simulink model "amplifierboard"  (R2020b)
settings: Solver=FixedStepDiscrete  StartTime=0.0  StopTime=2  FixedStep=0.01  RelTol=1e-3
InitFcn:
  | mbd_s32k_consistency_checks(bdroot(gcs));
undefined symbols (not defined in the file): AutoLowerVal, AutoRaiseVal, HoldVal, LED_En, LED_Off, LED_On, Logic_High, Logic_Low, LQFP, ManualLowerVal, ManualRaiseVal, PWRWNDW_CHDLCK, sC_bool_PWMEN, sC_cnt_FWSetting, sC_cnt_Mtr_DrvNo_HB, sC_cnt_PWMHB1to4, sC_cnt_PWMHB5to8, sC_cnt_TargetSlowRange, sC_pct_ManualMax, sC_pct_RampDwn, sC_pct_RampUp, sC_pct_StartPWM, sC_pct_Targetmax, SwitchPackRangeOffset, Threshold_Value, Tolerant_Time
libraries: mbd_s32k1xx_ec_toolbox x205, simulink x59, canmsglib x19, Filter x15, wndwcmd x3
(part 2 of 6)

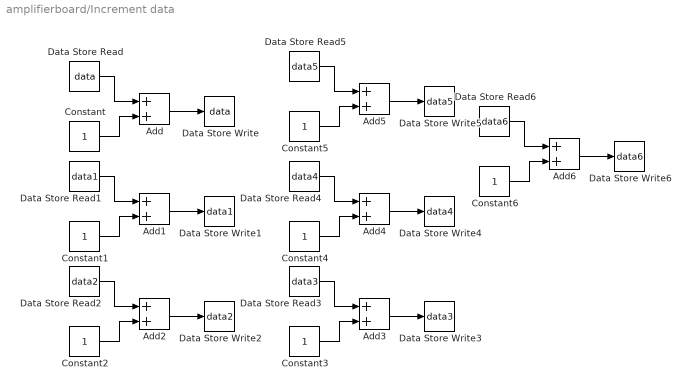
== system amplifierboard/Increment data ==
  Add{,1..6} (7 alike) : Sum
  Constant{,1..6} (7 alike) : Constant  OutDataTypeStr=uint8
  Data Store Read : DataStoreRead  DataStoreName=data
  Data Store Read1 : DataStoreRead  DataStoreName=data1
  Data Store Read2 : DataStoreRead  DataStoreName=data2
  Data Store Read3 : DataStoreRead  DataStoreName=data3
  Data Store Read4 : DataStoreRead  DataStoreName=data4
  Data Store Read5 : DataStoreRead  DataStoreName=data5
  Data Store Read6 : DataStoreRead  DataStoreName=data6
  Data Store Write : DataStoreWrite  DataStoreName=data
  Data Store Write1 : DataStoreWrite  DataStoreName=data1
  Data Store Write2 : DataStoreWrite  DataStoreName=data2
  Data Store Write3 : DataStoreWrite  DataStoreName=data3
  Data Store Write4 : DataStoreWrite  DataStoreName=data4
  Data Store Write5 : DataStoreWrite  DataStoreName=data5
  Data Store Write6 : DataStoreWrite  DataStoreName=data6
  wires:
  Add/1 -> Data Store Write/1
  Data Store Read/1 -> Add/1
  Constant/1 -> Add/2
  Constant1/1 -> Add1/2
  Add1/1 -> Data Store Write1/1
  Data Store Read1/1 -> Add1/1
  Constant2/1 -> Add2/2
  Add2/1 -> Data Store Write2/1
  Data Store Read2/1 -> Add2/1
  Data Store Read3/1 -> Add3/1
  Add3/1 -> Data Store Write3/1
  Constant3/1 -> Add3/2
  Constant4/1 -> Add4/2
  Add4/1 -> Data Store Write4/1
  Data Store Read4/1 -> Add4/1
  Data Store Read5/1 -> Add5/1
  Add5/1 -> Data Store Write5/1
  Constant5/1 -> Add5/2
  Constant6/1 -> Add6/2
  Add6/1 -> Data Store Write6/1
  Data Store Read6/1 -> Add6/1

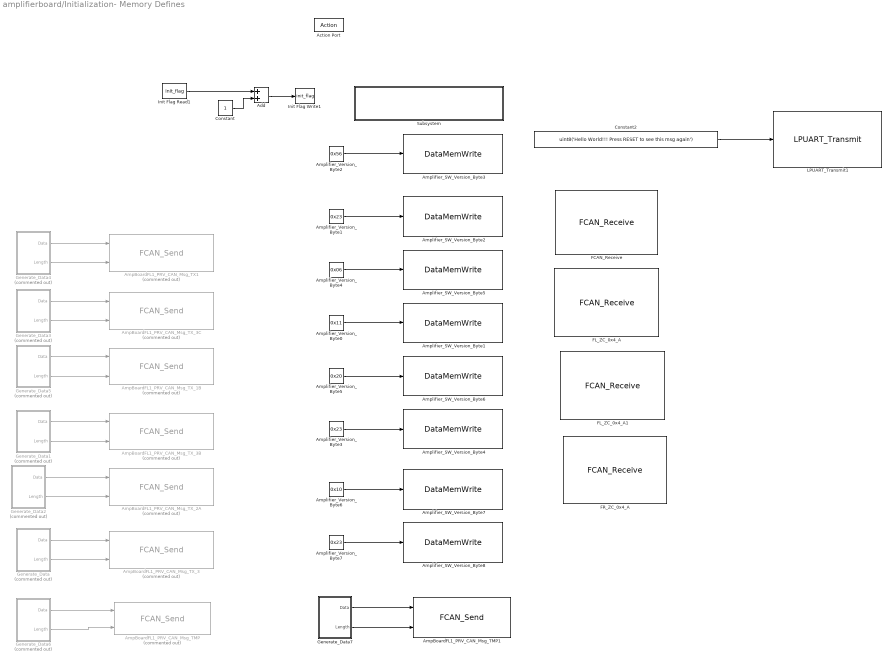
== system amplifierboard/Initialization- Memory Defines ==
  Action Port : ActionPort  InitializeStates=reset  ActionPortLabel=if(u1 <= 2)
  Add : Sum  AccumDataTypeStr=uint8  OutDataTypeStr=uint8
  AmpBoardFL1_PRV_CAN_Msg_TMP : mbd_s32k1xx_ec_toolbox/Communication Blocks/CAN Blocks/FCAN_Send  Commented=on  can_instance=1  can_mode=Non-blocking  can_timeout_ms=0  can_mb_idx=20  can_mb_init=On each call  show_id_input=off  can_extended_id=off  can_is_remote=off  can_id=113  show_adv_opts=on  can_fd_enable=off  can_enable_brs=off  can_fd_padding=0
  AmpBoardFL1_PRV_CAN_Msg_TMP1 : mbd_s32k1xx_ec_toolbox/Communication Blocks/CAN Blocks/FCAN_Send  can_instance=1  can_mode=Non-blocking  can_timeout_ms=0  can_mb_idx=9  can_mb_init=On each call  show_id_input=off  can_extended_id=off  can_is_remote=off  can_id=A9  show_adv_opts=on  can_fd_enable=off  can_enable_brs=off  can_fd_padding=0
  AmpBoardFL1_PRV_CAN_Msg_TX1 : mbd_s32k1xx_ec_toolbox/Communication Blocks/CAN Blocks/FCAN_Send  Priority=2  Commented=on  can_instance=1  can_mode=Non-blocking  can_timeout_ms=0  can_mb_idx=19  can_mb_init=On each call  show_id_input=off  can_extended_id=off  can_is_remote=off  can_id=6  show_adv_opts=off  can_fd_enable=off  can_enable_brs=off  can_fd_padding=0
  AmpBoardFL1_PRV_CAN_Msg_TX_1B : mbd_s32k1xx_ec_toolbox/Communication Blocks/CAN Blocks/FCAN_Send  Priority=2  Commented=on  can_instance=1  can_mode=Non-blocking  can_timeout_ms=0  can_mb_idx=17  can_mb_init=On each call  show_id_input=off  can_extended_id=off  can_is_remote=off  can_id=14  show_adv_opts=off  can_fd_enable=off  can_enable_brs=off  can_fd_padding=0
  AmpBoardFL1_PRV_CAN_Msg_TX_2A : mbd_s32k1xx_ec_toolbox/Communication Blocks/CAN Blocks/FCAN_Send  Priority=2  Commented=on  can_instance=1  can_mode=Non-blocking  can_timeout_ms=0  can_mb_idx=16  can_mb_init=On each call  show_id_input=off  can_extended_id=off  can_is_remote=off  can_id=20  show_adv_opts=off  can_fd_enable=off  can_enable_brs=off  can_fd_padding=0
  AmpBoardFL1_PRV_CAN_Msg_TX_3 : mbd_s32k1xx_ec_toolbox/Communication Blocks/CAN Blocks/FCAN_Send  Priority=2  Commented=on  can_instance=1  can_mode=Non-blocking  can_timeout_ms=0  can_mb_idx=14  can_mb_init=On each call  show_id_input=off  can_extended_id=off  can_is_remote=off  can_id=8  show_adv_opts=off  can_fd_enable=off  can_enable_brs=off  can_fd_padding=0
  AmpBoardFL1_PRV_CAN_Msg_TX_3B : mbd_s32k1xx_ec_toolbox/Communication Blocks/CAN Blocks/FCAN_Send  Priority=2  Commented=on  can_instance=1  can_mode=Non-blocking  can_timeout_ms=0  can_mb_idx=15  can_mb_init=On each call  show_id_input=off  can_extended_id=off  can_is_remote=off  can_id=13  show_adv_opts=off  can_fd_enable=off  can_enable_brs=off  can_fd_padding=0
  AmpBoardFL1_PRV_CAN_Msg_TX_3C : mbd_s32k1xx_ec_toolbox/Communication Blocks/CAN Blocks/FCAN_Send  Priority=2  Commented=on  can_instance=1  can_mode=Non-blocking  can_timeout_ms=0  can_mb_idx=18  can_mb_init=On each call  show_id_input=off  can_extended_id=off  can_is_remote=off  can_id=15  show_adv_opts=off  can_fd_enable=off  can_enable_brs=off  can_fd_padding=0
  Amplifier_SW_Version_Byte1 : mbd_s32k1xx_ec_toolbox/Utility Blocks/DataMemWrite  base=0x1FFFFFF0  offset=0x0003  ptr=uint8_t
  Amplifier_SW_Version_Byte2 : mbd_s32k1xx_ec_toolbox/Utility Blocks/DataMemWrite  base=0x1FFFFFF0  offset=0x0001  ptr=uint8_t
  Amplifier_SW_Version_Byte3 : mbd_s32k1xx_ec_toolbox/Utility Blocks/DataMemWrite  base=0x1FFFFFF0  offset=0x0000  ptr=uint8_t
  Amplifier_SW_Version_Byte4 : mbd_s32k1xx_ec_toolbox/Utility Blocks/DataMemWrite  base=0x1FFFFFF0  offset=0x0005  ptr=uint8_t
  Amplifier_SW_Version_Byte5 : mbd_s32k1xx_ec_toolbox/Utility Blocks/DataMemWrite  base=0x1FFFFFF0  offset=0x0002  ptr=uint8_t
  Amplifier_SW_Version_Byte6 : mbd_s32k1xx_ec_toolbox/Utility Blocks/DataMemWrite  base=0x1FFFFFF0  offset=0x0004  ptr=uint8_t
  Amplifier_SW_Version_Byte7 : mbd_s32k1xx_ec_toolbox/Utility Blocks/DataMemWrite  base=0x1FFFFFF0  offset=0x0006  ptr=uint8_t
  Amplifier_SW_Version_Byte8 : mbd_s32k1xx_ec_toolbox/Utility Blocks/DataMemWrite  base=0x1FFFFFF0  offset=0x0007  ptr=uint8_t
  Amplifier_Version_Byte0 : Constant  Value=0x11  OutDataTypeStr=uint8
  Amplifier_Version_Byte1 : Constant  Value=0x23  OutDataTypeStr=uint8
  Amplifier_Version_Byte2 : Constant  Value=0x56  OutDataTypeStr=uint8  LockScale=on
  Amplifier_Version_Byte3 : Constant  Value=0x23  OutDataTypeStr=uint8  LockScale=on
  Amplifier_Version_Byte4 : Constant  Value=0x06  OutDataTypeStr=uint8  LockScale=on
  Amplifier_Version_Byte5 : Constant  Value=0x20  OutDataTypeStr=uint8
  Amplifier_Version_Byte6 : Constant  Value=0x10  OutDataTypeStr=uint8
  Amplifier_Version_Byte7 : Constant  Value=0x23  OutDataTypeStr=uint8  LockScale=on
  Constant : Constant
  Constant2 : Constant  Value=uint8('Hello World!!! Press RESET to see this msg again')  SampleTime=-1
  FCAN_Receive : mbd_s32k1xx_ec_toolbox/Communication Blocks/CAN Blocks/FCAN_Receive  can_instance=1  can_mode=Non-blocking  can_timeout_ms=0  can_mb_idx=3  can_mb_init=Once  show_id_input=off  can_extended_id=off  can_is_remote=off  can_id=171  can_msg_mask=0  show_adv_opts=off  can_use_rxfifo=off  can_fd_enable=off
  FL_ZC_0x4_A : mbd_s32k1xx_ec_toolbox/Communication Blocks/CAN Blocks/FCAN_Receive  can_instance=1  can_mode=Non-blocking  can_timeout_ms=0  can_mb_idx=2  can_mb_init=Once  show_id_input=off  can_extended_id=off  can_is_remote=off  can_id=2  can_msg_mask=0  show_adv_opts=on  can_use_rxfifo=off  can_fd_enable=off
  FL_ZC_0x4_A1 : mbd_s32k1xx_ec_toolbox/Communication Blocks/CAN Blocks/FCAN_Receive  can_instance=1  can_mode=Non-blocking  can_timeout_ms=0  can_mb_idx=5  can_mb_init=Once  show_id_input=off  can_extended_id=off  can_is_remote=off  can_id=110  can_msg_mask=FF  show_adv_opts=on  can_use_rxfifo=off  can_fd_enable=off
  FR_ZC_0x4_A : mbd_s32k1xx_ec_toolbox/Communication Blocks/CAN Blocks/FCAN_Receive  can_instance=1  can_mode=Non-blocking  can_timeout_ms=0  can_mb_idx=6  can_mb_init=Once  show_id_input=off  can_extended_id=off  can_is_remote=off  can_id=110  can_msg_mask=FF  show_adv_opts=on  can_use_rxfifo=off  can_fd_enable=off
  Generate_Data : Subsystem  Commented=on
  Generate_Data1 : Subsystem  Commented=on
  Generate_Data2 : Subsystem  Commented=on
  Generate_Data3 : Subsystem  Commented=on
  Generate_Data4 : Subsystem  Commented=on
  Generate_Data5 : Subsystem  Commented=on
  Generate_Data6 : Subsystem  Commented=on
  Generate_Data7 : Subsystem
  Init Flag Read1 : DataStoreRead  DataStoreName=init_flag  DataStoreElements=init_flag
  Init Flag Write1 : DataStoreWrite  DataStoreName=init_flag  DataStoreElements=init_flag
  LPUART_Transmit1 : mbd_s32k1xx_ec_toolbox/Communication Blocks/UART Blocks/LPUART_Transmit  instance=2  transmit_mode=Non-blocking  timeout=500  number=off
  Subsystem : Subsystem
  wires:
  Amplifier_Version_Byte2/1 -> Amplifier_SW_Version_Byte3/1
  Amplifier_Version_Byte4/1 -> Amplifier_SW_Version_Byte5/1
  Amplifier_Version_Byte0/1 -> Amplifier_SW_Version_Byte1/1
  Amplifier_Version_Byte6/1 -> Amplifier_SW_Version_Byte7/1
  Amplifier_Version_Byte5/1 -> Amplifier_SW_Version_Byte6/1
  Amplifier_Version_Byte1/1 -> Amplifier_SW_Version_Byte2/1
  Amplifier_Version_Byte7/1 -> Amplifier_SW_Version_Byte8/1
  Amplifier_Version_Byte3/1 -> Amplifier_SW_Version_Byte4/1
  Generate_Data6/1(Data) -> AmpBoardFL1_PRV_CAN_Msg_TMP/1
  Generate_Data6/2(Length) -> AmpBoardFL1_PRV_CAN_Msg_TMP/2
  Generate_Data5/1(Data) -> AmpBoardFL1_PRV_CAN_Msg_TX_1B/1
  Generate_Data5/2(Length) -> AmpBoardFL1_PRV_CAN_Msg_TX_1B/2
  Generate_Data4/2(Length) -> AmpBoardFL1_PRV_CAN_Msg_TX1/2
  Generate_Data4/1(Data) -> AmpBoardFL1_PRV_CAN_Msg_TX1/1
  Generate_Data2/1(Data) -> AmpBoardFL1_PRV_CAN_Msg_TX_2A/1
  Generate_Data3/1(Data) -> AmpBoardFL1_PRV_CAN_Msg_TX_3C/1
  Generate_Data3/2(Length) -> AmpBoardFL1_PRV_CAN_Msg_TX_3C/2
  Generate_Data2/2(Length) -> AmpBoardFL1_PRV_CAN_Msg_TX_2A/2
  Generate_Data1/1(Data) -> AmpBoardFL1_PRV_CAN_Msg_TX_3B/1
  Generate_Data1/2(Length) -> AmpBoardFL1_PRV_CAN_Msg_TX_3B/2
  Generate_Data/2(Length) -> AmpBoardFL1_PRV_CAN_Msg_TX_3/2
  Generate_Data/1(Data) -> AmpBoardFL1_PRV_CAN_Msg_TX_3/1
  Add/1 -> Init Flag Write1/1
  Init Flag Read1/1 -> Add/1
  Constant/1 -> Add/2
  Constant2/1 -> LPUART_Transmit1/1
  Generate_Data7/2(Length) -> AmpBoardFL1_PRV_CAN_Msg_TMP1/2
  Generate_Data7/1(Data) -> AmpBoardFL1_PRV_CAN_Msg_TMP1/1

== system amplifierboard/Motor_Control ==
  Motor_Dir : Inport
  Constant{2..6} (5 alike) : Constant  Commented=on  Value=0  OutDataTypeStr=Inherit: Inherit via back propagation  SampleTime=-1
  Demux : Demux  Commented=on  Outputs=6
  FTM_PWM_Config_PTA11/PTA12/PTA13_PWM2/PWM3/PWM4 : mbd_s32k1xx_ec_toolbox/Motor Control Blocks/FTM Blocks/FTM_PWM_Config  Commented=on  ftmModule=1  ftmMode=Edge-Aligned PWM  ftmSourceClock=80 MHz  swcontrol_enable=off  chan0En=off  chan0Type=Complementary  chan2En=off  chan2Type=Complementary  chan4En=on  chan4Type=Independent  chan6En=on  chan6Type=Independent  ftmPwmUnits=Hz  outFrequency=20000  ftmPeriod=4000  ftmPrescaler=Divide by 1  deadtimeUnits=Nanoseconds  deadtimeNs=0  deadtimeTicks=0  deadtimePrescaler=Divide by 1  dutyCycleCh0=0  dutyCycleCh1=0  dutyCycleCh2=0  dutyCycleCh3=0  dutyCycleCh4=0  dutyCycleCh5=0  dutyCycleCh6=0.25  dutyCycleCh7=0.25  dutyCycleSim=off  startAfterInit=on  showAdvOpt=on  pinFtmCh0=PTB2: [FTM1_CH0 | FTM Channel]  pinFtmCh1=None  pinPolCh0=Active High  pinPolCh1=Active Low  outputComplem0=Main duplicated  outputLevel0=Low  outputLevel1=Low  pinFtmCh2=PTC14: [FTM1_CH2 | FTM Channel]  pinFtmCh3=None  pinPolCh2=Active High  pinPolCh3=Active Low  outputComplem2=Main duplicated  outputLevel2=Low  outputLevel3=Low  pinFtmCh4=PTD8: [FTM1_CH4 | FTM Channel]  pinFtmCh5=PTA11: [FTM1_CH5 | FTM Channel]  pinPolCh4=Active High  pinPolCh5=Active Low  outputComplem4=Main duplicated  outputLevel4=Low  outputLevel5=Low  pinFtmCh6=PTA12: [FTM1_CH6 | FTM Channel]  pinFtmCh7=PTA13: [FTM1_CH7 | FTM Channel]  pinPolCh6=Active High  pinPolCh7=Active High  outputComplem6=Main inverted  outputLevel6=Low  outputLevel7=Low  initTrigger=off  chTrigger0=off  chTrigger1=off  chTrigger2=off  chTrigger3=off  chTrigger4=off  chTrigger5=off  chTrigger6=off  chTrigger7=off  mcuTargetUpdate=on  pwmSyncTrg=Software trigger  pwmSyncHwRouting=TRGMUX_FTM7  pwmSyncTrg0=off  pwmSyncTrg1=off  pwmSyncTrg2=off  pwmSyncAutoClear=on  pwmSyncMinLoad=on  pwmSyncMaxLoad=on  pwmSyncInvert=System Clock  pwmSyncOutControl=System Clock  pwmSyncOutMask=System Clock  pwmSyncCounterInitial=System Clock  pwmSyncPoints=Update now  reloadEnable=off  reloadPriority=15  reloadHalfCycle=off  reloadHCR=0  reloadFrequency=0  chnMatch0=off  chnMatch1=off  chnMatch2=off  chnMatch3=off  chnMatch4=off  chnMatch5=off  chnMatch6=off  chnMatch7=off  pwmFaultProtection=off  pwmFaultInterrupt=off  pwmFaultClearing=Fault control disabled  pwmFaultPinState=Safe Value  pwmFaultFilterValue=0  pwmFaultPriority=15  fault_disen_0=off  fault_filter_0=off  fault_polarity_0=Active High  fault_disen_1=off  fault_filter_1=off  fault_polarity_1=Active high  fault_disen_2=off  fault_filter_2=off  fault_polarity_2=Active high  fault_disen_3=off  fault_filter_3=off  fault_polarity_3=Active high  fault_pin_0=None  fault_pin_1=None  fault_pin_2=None  fault_pin_3=None
  FTM_PWM_Config_PTA17/PTB17_PWM1/PWM5 : mbd_s32k1xx_ec_toolbox/Motor Control Blocks/FTM Blocks/FTM_PWM_Config  Commented=on  ftmModule=0  ftmMode=Edge-Aligned PWM  ftmSourceClock=80 MHz  swcontrol_enable=off  chan0En=off  chan0Type=Complementary  chan2En=off  chan2Type=Complementary  chan4En=on  chan4Type=Independent  chan6En=on  chan6Type=Complementary  ftmPwmUnits=Hz  outFrequency=20000  ftmPeriod=4000  ftmPrescaler=Divide by 1  deadtimeUnits=Nanoseconds  deadtimeNs=0  deadtimeTicks=0  deadtimePrescaler=Divide by 1  dutyCycleCh0=0  dutyCycleCh1=0  dutyCycleCh2=0  dutyCycleCh3=0  dutyCycleCh4=0  dutyCycleCh5=0  dutyCycleCh6=0.25  dutyCycleCh7=0.25  dutyCycleSim=off  startAfterInit=on  showAdvOpt=on  pinFtmCh0=PTB12: [FTM0_CH0 | FTM Channel]  pinFtmCh1=None  pinPolCh0=Active High  pinPolCh1=Active Low  outputComplem0=Main duplicated  outputLevel0=Low  outputLevel1=Low  pinFtmCh2=PTB14: [FTM0_CH2 | FTM Channel]  pinFtmCh3=None  pinPolCh2=Active High  pinPolCh3=Active Low  outputComplem2=Main duplicated  outputLevel2=Low  outputLevel3=Low  pinFtmCh4=PTB4: [FTM0_CH4 | FTM Channel]  pinFtmCh5=PTB17: [FTM0_CH5 | FTM Channel]  pinPolCh4=Active High  pinPolCh5=Active Low  outputComplem4=Main duplicated  outputLevel4=Low  outputLevel5=Low  pinFtmCh6=PTA17: [FTM0_CH6 | FTM Channel]  pinFtmCh7=None  pinPolCh6=Active High  pinPolCh7=Active Low  outputComplem6=Main duplicated  outputLevel6=Low  outputLevel7=Low  initTrigger=off  chTrigger0=off  chTrigger1=off  chTrigger2=off  chTrigger3=off  chTrigger4=off  chTrigger5=off  chTrigger6=off  chTrigger7=off  mcuTargetUpdate=on  pwmSyncTrg=Software trigger  pwmSyncHwRouting=TRGMUX_FTM7  pwmSyncTrg0=off  pwmSyncTrg1=off  pwmSyncTrg2=off  pwmSyncAutoClear=on  pwmSyncMinLoad=on  pwmSyncMaxLoad=on  pwmSyncInvert=System Clock  pwmSyncOutControl=System Clock  pwmSyncOutMask=System Clock  pwmSyncCounterInitial=System Clock  pwmSyncPoints=Update now  reloadEnable=off  reloadPriority=15  reloadHalfCycle=off  reloadHCR=0  reloadFrequency=0  chnMatch0=off  chnMatch1=off  chnMatch2=off  chnMatch3=off  chnMatch4=off  chnMatch5=off  chnMatch6=off  chnMatch7=off  pwmFaultProtection=off  pwmFaultInterrupt=off  pwmFaultClearing=Fault control disabled  pwmFaultPinState=Safe Value  pwmFaultFilterValue=0  pwmFaultPriority=15  fault_disen_0=off  fault_filter_0=off  fault_polarity_0=Active High  fault_disen_1=off  fault_filter_1=off  fault_polarity_1=Active high  fault_disen_2=off  fault_filter_2=off  fault_polarity_2=Active high  fault_disen_3=off  fault_filter_3=off  fault_polarity_3=Active high  fault_pin_0=None  fault_pin_1=None  fault_pin_2=None  fault_pin_3=None
  FTM_PWM_Config_PTB9/PTB10/PTB11_PWM6/PWM7/PWM8 : mbd_s32k1xx_ec_toolbox/Motor Control Blocks/FTM Blocks/FTM_PWM_Config  Commented=on  ftmModule=3  ftmMode=Center-Aligned PWM  ftmSourceClock=80 MHz  swcontrol_enable=off  chan0En=on  chan0Type=Independent  chan2En=on  chan2Type=Independent  chan4En=off  chan4Type=Independent  chan6En=off  chan6Type=Complementary  ftmPwmUnits=Hz  outFrequency=20000  ftmPeriod=4000  ftmPrescaler=Divide by 1  deadtimeUnits=Nanoseconds  deadtimeNs=0  deadtimeTicks=0  deadtimePrescaler=Divide by 1  dutyCycleCh0=0  dutyCycleCh1=0  dutyCycleCh2=0  dutyCycleCh3=0  dutyCycleCh4=0  dutyCycleCh5=0  dutyCycleCh6=0.25  dutyCycleCh7=0.25  dutyCycleSim=off  startAfterInit=on  showAdvOpt=on  pinFtmCh0=PTA2: [FTM3_CH0 | FTM Channel]  pinFtmCh1=PTB9: [FTM3_CH1 | FTM Channel]  pinPolCh0=Active High  pinPolCh1=Active Low  outputComplem0=Main duplicated  outputLevel0=Low  outputLevel1=Low  pinFtmCh2=PTB10: [FTM3_CH2 | FTM Channel]  pinFtmCh3=PTB11: [FTM3_CH3 | FTM Channel]  pinPolCh2=Active High  pinPolCh3=Active Low  outputComplem2=Main duplicated  outputLevel2=Low  outputLevel3=Low  pinFtmCh4=PTC10: [FTM3_CH4 | FTM Channel]  pinFtmCh5=None  pinPolCh4=Active Low  pinPolCh5=Active Low  outputComplem4=Main inverted  outputLevel4=Low  outputLevel5=Low  pinFtmCh6=PTC12: [FTM3_CH6 | FTM Channel]  pinFtmCh7=None  pinPolCh6=Active High  pinPolCh7=Active Low  outputComplem6=Main duplicated  outputLevel6=Low  outputLevel7=Low  initTrigger=off  chTrigger0=off  chTrigger1=off  chTrigger2=off  chTrigger3=off  chTrigger4=off  chTrigger5=off  chTrigger6=off  chTrigger7=off  mcuTargetUpdate=on  pwmSyncTrg=Software trigger  pwmSyncHwRouting=TRGMUX_FTM7  pwmSyncTrg0=off  pwmSyncTrg1=off  pwmSyncTrg2=off  pwmSyncAutoClear=on  pwmSyncMinLoad=on  pwmSyncMaxLoad=on  pwmSyncInvert=System Clock  pwmSyncOutControl=System Clock  pwmSyncOutMask=System Clock  pwmSyncCounterInitial=System Clock  pwmSyncPoints=Update now  reloadEnable=off  reloadPriority=15  reloadHalfCycle=off  reloadHCR=0  reloadFrequency=0  chnMatch0=off  chnMatch1=off  chnMatch2=off  chnMatch3=off  chnMatch4=off  chnMatch5=off  chnMatch6=off  chnMatch7=off  pwmFaultProtection=off  pwmFaultInterrupt=off  pwmFaultClearing=Fault control disabled  pwmFaultPinState=Safe Value  pwmFaultFilterValue=0  pwmFaultPriority=15  fault_disen_0=off  fault_filter_0=off  fault_polarity_0=Active High  fault_disen_1=off  fault_filter_1=off  fault_polarity_1=Active high  fault_disen_2=off  fault_filter_2=off  fault_polarity_2=Active high  fault_disen_3=off  fault_filter_3=off  fault_polarity_3=Active high  fault_pin_0=None  fault_pin_1=None  fault_pin_2=None  fault_pin_3=None
  From : From  Commented=on  GotoTag=PWM1
  From1 : From  Commented=on  GotoTag=PWM2
  From2 : From  Commented=on  GotoTag=PWM3
  From3 : From  Commented=on  GotoTag=PWM4
  From4 : From  Commented=on  GotoTag=PWM5
  From5 : From  Commented=on  GotoTag=PWM6
  Goto17 : Goto  Commented=on  GotoTag=PWM2
  Goto34 : Goto  Commented=on  GotoTag=PWM3
  Goto35 : Goto  Commented=on  GotoTag=PWM4
  Goto36 : Goto  Commented=on  GotoTag=PWM5
  Goto37 : Goto  Commented=on  GotoTag=PWM6
  Goto6 : Goto  Commented=on  GotoTag=PWM1
  Motor_Control : Subsystem
  Subsystem : Subsystem  Commented=on
  8718_FailSafe : Outport
  MotorDriverState : Outport  Port=2
  wires:
  Motor_Dir/1 -> Subsystem/1(cMM_aV_int_MotorDir1), Motor_Control/1(cMM_aV_int_MotorDir)
  Constant5/1 -> FTM_PWM_Config_PTB9/PTB10/PTB11_PWM6/PWM7/PWM8/1
  Demux/1 -> Goto6/1
  Demux/3 -> Goto34/1
  From4/1 -> FTM_PWM_Config_PTA17/PTB17_PWM1/PWM5/2
  From/1 -> FTM_PWM_Config_PTA17/PTB17_PWM1/PWM5/3
  Constant4/1 -> FTM_PWM_Config_PTA11/PTA12/PTA13_PWM2/PWM3/PWM4/1
  Constant6/1 -> FTM_PWM_Config_PTB9/PTB10/PTB11_PWM6/PWM7/PWM8/3
  Demux/2 -> Goto17/1
  Demux/4 -> Goto35/1
  Constant2/1 -> FTM_PWM_Config_PTA17/PTB17_PWM1/PWM5/1
  From3/1 -> FTM_PWM_Config_PTA11/PTA12/PTA13_PWM2/PWM3/PWM4/4
  From1/1 -> FTM_PWM_Config_PTA11/PTA12/PTA13_PWM2/PWM3/PWM4/2
  Demux/5 -> Goto36/1
  From5/1 -> FTM_PWM_Config_PTB9/PTB10/PTB11_PWM6/PWM7/PWM8/2
  Demux/6 -> Goto37/1
  Subsystem/1(aV_pct_PWMOut1) -> Demux/1
  From2/1 -> FTM_PWM_Config_PTA11/PTA12/PTA13_PWM2/PWM3/PWM4/3
  Constant3/1 -> FTM_PWM_Config_PTB9/PTB10/PTB11_PWM6/PWM7/PWM8/4
  Motor_Control/1(8718_FailSafe) -> 8718_FailSafe/1
  Motor_Control/2(MotorDriverState) -> MotorDriverState/1

== system amplifierboard/TC1047A_Module ==
  ADC_Start : mbd_s32k1xx_ec_toolbox/Motor Control Blocks/ADC Blocks/ADC_Start  Priority=2  instance=1  adc_r=A  adc_chan=PTA15: [ADC1_SE12 | ADC Single Ended Input]  aien=off  mcuTargetUpdate=on
  temperature_conversion : Subsystem
  AmpBoard_PRV_CAN_Msg_TX_TMP : Outport
  wires:
  ADC_Start/1 -> temperature_conversion/1(In1)
  temperature_conversion/1(AmpBoard_PRV_CAN_Msg_TX_TMP) -> AmpBoard_PRV_CAN_Msg_TX_TMP/1

== system amplifierboard/CAN_Pack_And_Send/CAN_Msg ==
  CAN_Msg : Inport
  Action Port : ActionPort  ActionPortLabel=if(u1 == 0 & u2 == 1)
  Bus Selector2 : BusSelector  OutputSignals=Data,Length
  FCAN_Send2 : mbd_s32k1xx_ec_toolbox/Communication Blocks/CAN Blocks/FCAN_Send  can_instance=1  can_mode=Non-blocking  can_timeout_ms=0  can_mb_idx=16  can_mb_init=On each call  show_id_input=off  can_extended_id=off  can_is_remote=off  can_id=8  show_adv_opts=on  can_fd_enable=off  can_enable_brs=off  can_fd_padding=0
  wires:
  Bus Selector2/2 -> FCAN_Send2/2  "<Length>"
  Bus Selector2/1 -> FCAN_Send2/1  "<Data>"
  CAN_Msg/1 -> Bus Selector2/1

== system amplifierboard/CAN_Pack_And_Send/CAN_Msg1 ==
  CAN_Msg : Inport
  Action Port : ActionPort  ActionPortLabel=if(u1 == 0 & u2 == 1)
  Bus Selector2 : BusSelector  OutputSignals=Data,Length
  FCAN_Send2 : mbd_s32k1xx_ec_toolbox/Communication Blocks/CAN Blocks/FCAN_Send  can_instance=1  can_mode=Non-blocking  can_timeout_ms=0  can_mb_idx=17  can_mb_init=On each call  show_id_input=off  can_extended_id=off  can_is_remote=off  can_id=13  show_adv_opts=on  can_fd_enable=off  can_enable_brs=off  can_fd_padding=0
  wires:
  Bus Selector2/2 -> FCAN_Send2/2  "<Length>"
  Bus Selector2/1 -> FCAN_Send2/1  "<Data>"
  CAN_Msg/1 -> Bus Selector2/1

== system amplifierboard/CAN_Pack_And_Send/CAN_Msg2 ==
  CAN_Msg : Inport
  Action Port : ActionPort  ActionPortLabel=if(u1 == 0 & u2 == 1)
  Bus Selector2 : BusSelector  OutputSignals=Data,Length
  FCAN_Send2 : mbd_s32k1xx_ec_toolbox/Communication Blocks/CAN Blocks/FCAN_Send  can_instance=1  can_mode=Non-blocking  can_timeout_ms=0  can_mb_idx=18  can_mb_init=On each call  show_id_input=off  can_extended_id=off  can_is_remote=off  can_id=7  show_adv_opts=on  can_fd_enable=off  can_enable_brs=off  can_fd_padding=0
  wires:
  CAN_Msg/1 -> Bus Selector2/1
  Bus Selector2/1 -> FCAN_Send2/1  "<Data>"
  Bus Selector2/2 -> FCAN_Send2/2  "<Length>"

== system amplifierboard/CAN_Pack_And_Send/CAN_Msg3 ==
  CAN_Msg : Inport
  Action Port : ActionPort  ActionPortLabel=if(u1 == 0 & u2 == 1)
  Bus Selector2 : BusSelector  OutputSignals=Data,Length
  FCAN_Send2 : mbd_s32k1xx_ec_toolbox/Communication Blocks/CAN Blocks/FCAN_Send  can_instance=1  can_mode=Non-blocking  can_timeout_ms=0  can_mb_idx=21  can_mb_init=On each call  show_id_input=off  can_extended_id=off  can_is_remote=off  can_id=15  show_adv_opts=on  can_fd_enable=off  can_enable_brs=off  can_fd_padding=0
  wires:
  Bus Selector2/2 -> FCAN_Send2/2  "<Length>"
  Bus Selector2/1 -> FCAN_Send2/1  "<Data>"
  CAN_Msg/1 -> Bus Selector2/1

== system amplifierboard/CAN_Pack_And_Send/CAN_Msg_temp ==
  CAN_Msg : Inport
  Action Port : ActionPort  ActionPortLabel=if(u1 == 0 & u2 == 1)
  AmpBoardFL1_PRV_CAN_Msg_TMP : mbd_s32k1xx_ec_toolbox/Communication Blocks/CAN Blocks/FCAN_Send  can_instance=1  can_mode=Non-blocking  can_timeout_ms=0  can_mb_idx=19  can_mb_init=On each call  show_id_input=off  can_extended_id=off  can_is_remote=off  can_id=113  show_adv_opts=on  can_fd_enable=off  can_enable_brs=off  can_fd_padding=0
  Bus Selector2 : BusSelector  OutputSignals=Data,Length
  wires:
  Bus Selector2/2 -> AmpBoardFL1_PRV_CAN_Msg_TMP/2  "<Length>"
  Bus Selector2/1 -> AmpBoardFL1_PRV_CAN_Msg_TMP/1  "<Data>"
  CAN_Msg/1 -> Bus Selector2/1

== system amplifierboard/CAN_Pack_And_Send/MtrSts ==
  CAN_Msg : Inport
  Action Port : ActionPort  ActionPortLabel=if(u1 == 0 & u2 == 1)
  Bus Selector2 : BusSelector  OutputSignals=Data,Length
  FCAN_Send2 : mbd_s32k1xx_ec_toolbox/Communication Blocks/CAN Blocks/FCAN_Send  can_instance=1  can_mode=Non-blocking  can_timeout_ms=0  can_mb_idx=20  can_mb_init=On each call  show_id_input=off  can_extended_id=off  can_is_remote=off  can_id=6  show_adv_opts=on  can_fd_enable=off  can_enable_brs=off  can_fd_padding=0
  wires:
  Bus Selector2/2 -> FCAN_Send2/2  "<Length>"
  Bus Selector2/1 -> FCAN_Send2/1  "<Data>"
  CAN_Msg/1 -> Bus Selector2/1

== system amplifierboard/CAN_Pack_And_Send/MtrSts1 ==
  CAN_Msg : Inport
  Action Port : ActionPort  ActionPortLabel=if(u1 == 0 & u2 == 1)
  Bus Selector2 : BusSelector  OutputSignals=Data,Length
  FCAN_Send2 : mbd_s32k1xx_ec_toolbox/Communication Blocks/CAN Blocks/FCAN_Send  can_instance=1  can_mode=Non-blocking  can_timeout_ms=0  can_mb_idx=22  can_mb_init=On each call  show_id_input=off  can_extended_id=off  can_is_remote=off  can_id=14  show_adv_opts=on  can_fd_enable=off  can_enable_brs=off  can_fd_padding=0
  wires:
  CAN_Msg/1 -> Bus Selector2/1
  Bus Selector2/1 -> FCAN_Send2/1  "<Data>"
  Bus Selector2/2 -> FCAN_Send2/2  "<Length>"

== system amplifierboard/CAN_Pack_And_Send/PsngrWndwCntDetect ==
  SwitchCount : Inport
  SwtchPosDetect : Subsystem  AncestorBlock=wndwenble_2020b/WndwCntDetect/SwtchPosDetect
  AvgCount : Outport
  wires:
  SwtchPosDetect/1(AvgCount) -> AvgCount/1  "AvgCount"
  SwitchCount/1 -> SwtchPosDetect/1(SwitchCount)  "SwitchCount"

== system amplifierboard/CAN_Pack_And_Send/RLWndwCntDetect ==
  SwitchCount : Inport
  SwtchPosDetect : Subsystem  AncestorBlock=wndwenble_2020b/WndwCntDetect/SwtchPosDetect
  AvgCount : Outport
  wires:
  SwtchPosDetect/1(AvgCount) -> AvgCount/1  "AvgCount"
  SwitchCount/1 -> SwtchPosDetect/1(SwitchCount)  "SwitchCount"

== system amplifierboard/CAN_Pack_And_Send/RRWndwCntDetect ==
  SwitchCount : Inport
  SwtchPosDetect : Subsystem  AncestorBlock=wndwenble_2020b/WndwCntDetect/SwtchPosDetect
  AvgCount : Outport
  wires:
  SwtchPosDetect/1(AvgCount) -> AvgCount/1  "AvgCount"
  SwitchCount/1 -> SwtchPosDetect/1(SwitchCount)  "SwitchCount"

== system amplifierboard/CAN_Receive_And_Unpack/FL_Wndw ==
  Data : Inport
  Action Port : ActionPort  ActionPortLabel=if(u1 == 0)
  CAN Pack2 : canmsglib/CAN Pack  MsgList=(none)  MsgName=POWER_WINDOW_CTRL_DR  MsgIDType=Standard (11-bit identifier)  MsgIdentifier=0x110  MsgLength=8  Remote=off  ApplyMinMax=off  BusOutput=off  SignalInfo={}
      settings: SourceProductBaseCode=ME,XP,VN  DataFormat=raw data
  CAN Unpack2 : canmsglib/CAN Unpack  CANdbFile=C:\Work\repos\GenericAB\poc_communication_matrix\Zonal_Controller_FL\DBC_ZC_FL_CAN_3.dbc  MsgList=POWER_WINDOW_CTRL_DR  MsgName=POWER_WINDOW_CTRL_DR  MsgIDType=Standard (11-bit identifier)  MsgIdentifier=272  MsgLength=8  SignalInfo={'ChildLockCommandRL','29','2','BE','unsigned','Standard','0','1','0','0','3';'DriverWindowOperationPermission','16','2','BE','unsigned','Standard','0','1','0','0','3';'DrvWindowCommand','18','3','BE','unsigned','Standard','0','1','0','0','7';'ExternalTempCommandDriver','40','16','BE','unsigned','Standard','0','0.5','-40','-40','125';'ExternalTemperatureFailStsDriver','21','2','BE','unsigned','Standard','0','1','0','0','3';'RearLeftWindowCommand','26','3','BE','unsigned','Standard','0','1','0','0','7';'RearLeftWndOprnPerm','24','2','BE','unsigned','Standard','0','1','0','0','3'}  IDPort=off  TimestampPort=off  ErrorPort=off  RemotePort=off  LengthPort=off  StatusPort=off  ApplyMinMax=off
      settings: SourceProductBaseCode=ME,XP,VN  DataFormat=CANdb specified signals
  Terminator{,1..5} (6 alike) : Terminator
  WndwCmd : wndwcmd/WndwCmd  SystemSampleTime=-1  VariantActivationTime=update diagram  Latency=0  AutoFrameSizeCalculation=off
  RLWindwCmndCls : Outport
  RLWindwCmndOpn : Outport  Port=2
  wires:
  WndwCmd/1 -> RLWindwCmndCls/1
  CAN Unpack2/7 -> Terminator5/1
  WndwCmd/2 -> RLWindwCmndOpn/1
  CAN Unpack2/6 -> WndwCmd/1
  CAN Unpack2/2 -> Terminator1/1
  CAN Unpack2/1 -> Terminator/1
  CAN Pack2/1 -> CAN Unpack2/1
  Data/1 -> CAN Pack2/1
  CAN Unpack2/4 -> Terminator3/1
  CAN Unpack2/3 -> Terminator2/1
  CAN Unpack2/5 -> Terminator4/1

== system amplifierboard/CAN_Receive_And_Unpack/FR_Wndw ==
  Data : Inport
  Action Port : ActionPort  ActionPortLabel=if(u1 == 0)
  CAN Pack2 : canmsglib/CAN Pack  MsgList=(none)  MsgName=POWER_WINDOW_CTRL_PS  MsgIDType=Standard (11-bit identifier)  MsgIdentifier=0x110  MsgLength=8  Remote=off  ApplyMinMax=off  BusOutput=off  SignalInfo={}
      settings: SourceProductBaseCode=ME,XP,VN  DataFormat=raw data
  CAN Unpack2 : canmsglib/CAN Unpack  CANdbFile=C:\Work\repos\GenericAB\poc_communication_matrix\Zonal_Controller_FR\DBC_ZC_FR_CAN_4.dbc  MsgList=POWER_WINDOW_CTRL_PS  MsgName=POWER_WINDOW_CTRL_PS  MsgIDType=Standard (11-bit identifier)  MsgIdentifier=272  MsgLength=8  SignalInfo={'ChildLockCommandRR','29','2','BE','unsigned','Standard','0','1','0','0','3';'ExternalTempCommandPassenger','40','16','BE','unsigned','Standard','0','0.5','-40','-40','125';'ExternalTemperatureFailStsPsngr','21','2','BE','unsigned','Standard','0','1','0','0','3';'FrontPsngrWindowCommand','18','3','BE','unsigned','Standard','0','1','0','0','7';'FrontPsngrWndOprnPerm','16','2','BE','unsigned','Standard','0','1','0','0','3';'RearRightWindowCommand','26','3','BE','unsigned','Standard','0','1','0','0','7';'RearRightWndOprnPerm','24','2','BE','unsigned','Standard','0','1','0','0','3'}  IDPort=off  TimestampPort=off  ErrorPort=off  RemotePort=off  LengthPort=off  StatusPort=off  ApplyMinMax=off
      settings: SourceProductBaseCode=ME,XP,VN  DataFormat=CANdb specified signals
  Terminator{,1..2,4..5} (5 alike) : Terminator
  WndwCmd : wndwcmd/WndwCmd  SystemSampleTime=-1  VariantActivationTime=update diagram  Latency=0  AutoFrameSizeCalculation=off
  WndwCmd1 : wndwcmd/WndwCmd  SystemSampleTime=-1  VariantActivationTime=update diagram  Latency=0  AutoFrameSizeCalculation=off
  FPsngrWindwCmndCls : Outport
  FPsngrWindwCmndOpn : Outport  Port=2
  RRWindwCmndCls : Outport  Port=3
  RRWindwCmndOpn : Outport  Port=4
  wires:
  WndwCmd/1 -> RRWindwCmndCls/1
  CAN Unpack2/7 -> Terminator5/1
  WndwCmd/2 -> RRWindwCmndOpn/1
  CAN Unpack2/6 -> WndwCmd/1
  CAN Unpack2/2 -> Terminator1/1
  CAN Unpack2/1 -> Terminator/1
  CAN Pack2/1 -> CAN Unpack2/1
  Data/1 -> CAN Pack2/1
  CAN Unpack2/4 -> WndwCmd1/1
  CAN Unpack2/3 -> Terminator2/1
  CAN Unpack2/5 -> Terminator4/1
  WndwCmd1/1 -> FPsngrWindwCmndCls/1
  WndwCmd1/2 -> FPsngrWindwCmndOpn/1

== system amplifierboard/CAN_Receive_And_Unpack/If Action Subsystem2 ==
  Data : Inport
  Action Port : ActionPort  ActionPortLabel=if(u1 == 0)
  CAN Pack1 : canmsglib/CAN Pack  MsgList=(none)  MsgName=AB_Door_FL_PRV_CAN_Msg_RX1  MsgIDType=Standard (11-bit identifier)  MsgIdentifier=3  MsgLength=8  Remote=off  ApplyMinMax=off  BusOutput=off  SignalInfo={}
      settings: SourceProductBaseCode=ME,XP,VN  DataFormat=raw data
  CAN Unpack1 : canmsglib/CAN Unpack  CANdbFile=C:\Work\repos\GenericAB\poc_communication_matrix\Zonal_Controller_FL\DBC_ZC_FL_CAN_3.dbc  MsgList=AB_Door_FL_PRV_CAN_Msg_RX2  MsgName=AB_Door_FL_PRV_CAN_Msg_RX2  MsgIDType=Standard (11-bit identifier)  MsgIdentifier=3  MsgLength=8  SignalInfo={'AmpBoard_PRV_CAN_Msg_RX2_Alive','8','4','BE','unsigned','Standard','0','1','0','0','14';'AmpBoard_PRV_CAN_Msg_RX2_CRC','0','8','BE','unsigned','Standard','0','1','0','0','255';'Speed_Motor_01','16','8','BE','unsigned','Standard','0','1','0','0','255';'Speed_Motor_02','24','8','BE','unsigned','Standard','0','1','0','0','255';'Speed_Motor_03','32','8','BE','unsigned','Standard','0','1','0','0','255';'Speed_Motor_04','40','8','BE','unsigned','Standard','0','1','0','0','255';'Speed_Motor_05','48','8','BE','unsigned','Standard','0','1','0','0','255';'Speed_Motor_06','56','8','BE','unsigned','Standard','0','1','0','0','255'}  IDPort=off  TimestampPort=off  ErrorPort=off  RemotePort=off  LengthPort=off  StatusPort=off  ApplyMinMax=off
      settings: SourceProductBaseCode=ME,XP,VN  DataFormat=CANdb specified signals
  Terminator{1..8} (8 alike) : Terminator
  wires:
  Data/1 -> CAN Pack1/1
  CAN Unpack1/4 -> Terminator3/1
  CAN Unpack1/5 -> Terminator4/1
  CAN Unpack1/6 -> Terminator5/1
  CAN Unpack1/2 -> Terminator1/1
  CAN Unpack1/1 -> Terminator8/1
  CAN Unpack1/3 -> Terminator2/1
  CAN Unpack1/7 -> Terminator6/1
  CAN Pack1/1 -> CAN Unpack1/1
  CAN Unpack1/8 -> Terminator7/1

== system amplifierboard/CAN_Receive_And_Unpack/If Action Subsystem3 ==
  Data : Inport
  Action Port : ActionPort  ActionPortLabel=if(u1 == 0)
  CAN Pack1 : canmsglib/CAN Pack  MsgList=(none)  MsgName=AB_Door_FL_PRV_CAN_Msg_RX3  MsgIDType=Standard (11-bit identifier)  MsgIdentifier=4  MsgLength=8  Remote=off  ApplyMinMax=off  BusOutput=off  SignalInfo={}
      settings: SourceProductBaseCode=ME,XP,VN  DataFormat=raw data
  CAN Unpack1 : canmsglib/CAN Unpack  CANdbFile=C:\Work\repos\GenericAB\poc_communication_matrix\Zonal_Controller_FL\DBC_ZC_FL_CAN_3.dbc  MsgList=AB_Door_FL_PRV_CAN_Msg_RX3  MsgName=AB_Door_FL_PRV_CAN_Msg_RX3  MsgIDType=Standard (11-bit identifier)  MsgIdentifier=4  MsgLength=8  SignalInfo={'AmpBoard_PRV_CAN_Msg_RX3_Alive','8','4','BE','unsigned','Standard','0','1','0','0','14';'AmpBoard_PRV_CAN_Msg_RX3_CRC','0','8','BE','unsigned','Standard','0','1','0','0','255';'PWM_1','24','8','BE','unsigned','Standard','0','1','0','0','255';'PWM_2','32','8','BE','unsigned','Standard','0','1','0','0','255';'PWM_3','40','8','BE','unsigned','Standard','0','1','0','0','255';'PWM_4','48','8','BE','unsigned','Standard','0','1','0','0','255';'PWM_5','56','8','BE','unsigned','Standard','0','1','0','0','255';'PWM_Enable_Mask','16','5','BE','unsigned','Standard','0','1','0','0','31'}  IDPort=off  TimestampPort=off  ErrorPort=off  RemotePort=off  LengthPort=off  StatusPort=off  ApplyMinMax=off
      settings: SourceProductBaseCode=ME,XP,VN  DataFormat=CANdb specified signals
  Terminator{1..8} (8 alike) : Terminator
  wires:
  CAN Pack1/1 -> CAN Unpack1/1
  CAN Unpack1/5 -> Terminator4/1
  CAN Unpack1/8 -> Terminator7/1
  CAN Unpack1/2 -> Terminator1/1
  CAN Unpack1/4 -> Terminator3/1
  CAN Unpack1/3 -> Terminator2/1
  Data/1 -> CAN Pack1/1
  CAN Unpack1/7 -> Terminator6/1
  CAN Unpack1/6 -> Terminator5/1
  CAN Unpack1/1 -> Terminator8/1

== system amplifierboard/CAN_Receive_And_Unpack/Subsystem ==
  Data1 : Inport
  TimeStamp : Inport  Port=2
  CAN Pack1 : canmsglib/CAN Pack  MsgList=(none)  MsgName=AmpBoardFL1_PRV_CAN_Msg_RX1  MsgIDType=Standard (11-bit identifier)  MsgIdentifier=171  MsgLength=8  Remote=off  ApplyMinMax=off  BusOutput=off  SignalInfo={ 'Amplifier_Identifier', '0', '8', 'LE', 'unsigned', 'Standard', '0', '1', '0', '-Inf', 'Inf'; 'Reserved', '8', '54', 'LE', 'signed', 'Standard', '0', '1', '0', '-Inf', 'Inf' }
      settings: SourceProductBaseCode=ME,XP,VN  DataFormat=raw data
  CAN Unpack1 : canmsglib/CAN Unpack  MsgList=(none)  MsgName=CAN Msg  MsgIDType=Standard (11-bit identifier)  MsgIdentifier=171  MsgLength=8  SignalInfo={ 'ProtocolControlInfo', '0', '8', 'LE', 'unsigned', 'Standard', '0', '1', '0', '-Inf', 'Inf'; 'ServiceID', '8', '8', 'LE', 'unsigned', 'Standard', '0', '1', '0', '-Inf', 'Inf'; 'ServiceByte0', '16', '8', 'LE', 'unsigned', 'Standard', '0', '1', '0', '-Inf', 'Inf'; 'ServiceByte1', '24', '8', 'LE', 'unsigned', 'Standard', '0', '1', '0', '-Inf', 'Inf'; 'ServiceByte2', '32', '8', 'LE', 'unsigned', 'Standard', '0', '1', '0', '-Inf', 'Inf'; 'ServiceBtye3', '40', '8', 'LE', 'unsigned', 'Standard', '0', '1', '0', '-Inf', 'Inf' }  IDPort=off  TimestampPort=off  ErrorPort=off  RemotePort=off  LengthPort=off  StatusPort=off  ApplyMinMax=off
      settings: SourceProductBaseCode=ME,XP,VN
  Chart : Stateflow chart  TreatAsAtomicUnit=on
      settings: MinAlgLoopOccurrences=on
  Data Store Memory2 : DataStoreMemory  DataStoreName=PreviousTimeStamp  ReadBeforeWriteMsg=warning  WriteAfterWriteMsg=warning  WriteAfterReadMsg=warning  ShowAdditionalParam=off
  Data Store Memory3 : DataStoreMemory  DataStoreName=NewMsgRXed  ReadBeforeWriteMsg=warning  WriteAfterWriteMsg=warning  WriteAfterReadMsg=warning  ShowAdditionalParam=off  OutDataTypeStr=boolean
  Data Store Read2 : DataStoreRead  DataStoreName=PreviousTimeStamp
  Data Store Read3 : DataStoreRead  DataStoreName=NewMsgRXed
  If Action Subsystem1 : Subsystem  TreatAsAtomicUnit=on
  If Action Subsystem2 : Subsystem  TreatAsAtomicUnit=on
  If1 : If  NumInputs=3  IfExpression=(u1 ~= u2) | ( u3 == 1)
  LPSPI_Config 2 : mbd_s32k1xx_ec_toolbox/Communication Blocks/SPI Blocks/LPSPI_Config   Priority=0  InstanceNumber=0  Role=Master  BaudRate=10000  ShowAdvanced=on  sin=PTD16: [LPSPI0_SIN | LPSPI Serial Data Input]  sout=PTB4: [LPSPI0_SOUT | LPSPI Serial Data Output]  sck=PTD15: [LPSPI0_SCK | LPSPI Serial Clock I/O]  pcs0=PTB5: [LPSPI0_PCS0 | Peripheral Chip Select 0]  pcs1=None  pcs2=None  pcs3=None  CPHA=1  CPOL=0  BitOrder=MSB first  TransferSize=8  WhichPCS=0  PCSPol=ActiveLow  ContinuousTransfer=on
  StateFlowState : Outport
  CAN_Msg_PCI : Outport  Port=2
  LIN_Status : Outport  Port=3
  wires:
  CAN Unpack1/4 -> Chart/3(ServiceByte1)
  CAN Unpack1/5 -> Chart/4(ServiceByte2)
  CAN Pack1/1 -> CAN Unpack1/1
  Data1/1 -> CAN Pack1/1
  Chart/1(StateFlowState) -> StateFlowState/1
  CAN Unpack1/2 -> Chart/1(ServiceID)
  CAN Unpack1/3 -> Chart/2(ServiceByte0)
  CAN Unpack1/1 -> CAN_Msg_PCI/1
  Chart/2(ContinueStateProcessing) -> If1/3
  Data Store Read2/1 -> If1/1
  TimeStamp/1 -> If Action Subsystem1/1(TImeStamp), If1/2
  If1/1 -> If Action Subsystem1/Action
  Data Store Read3/1 -> Chart/6(NewMsgRXed)
  If1/2 -> If Action Subsystem2/Action
  CAN Unpack1/6 -> Chart/5(ServiceByte3)
  Chart/3(LIN_Status) -> LIN_Status/1

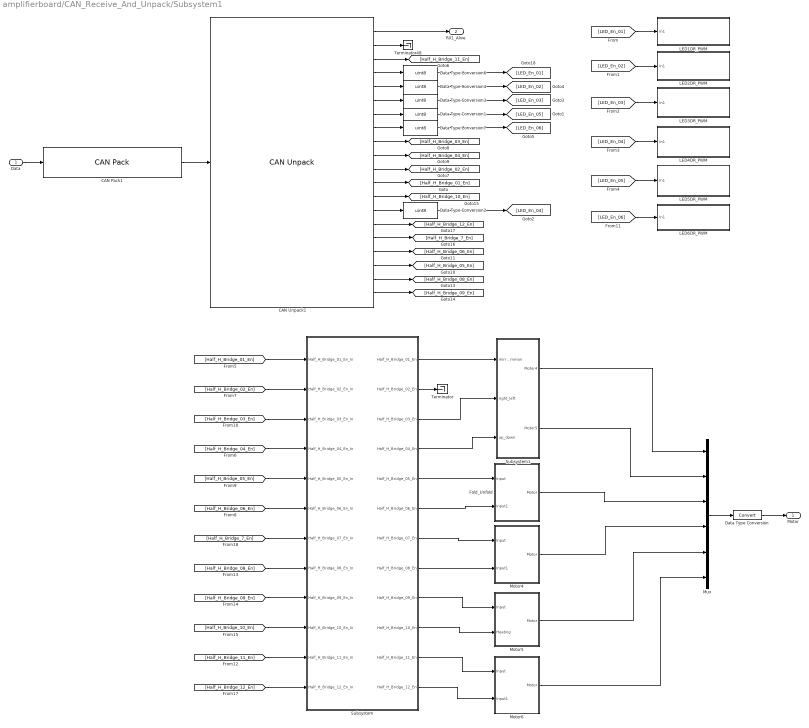
== system amplifierboard/CAN_Receive_And_Unpack/Subsystem1 ==
  Data : Inport
  CAN Pack1 : canmsglib/CAN Pack  MsgList=(none)  MsgName=AB_Door_FL_PRV_CAN_Msg_RX1  MsgIDType=Standard (11-bit identifier)  MsgIdentifier=2  MsgLength=8  Remote=off  ApplyMinMax=off  BusOutput=off  SignalInfo={}
      settings: SourceProductBaseCode=ME,XP,VN  DataFormat=raw data
  CAN Unpack1 : canmsglib/CAN Unpack  CANdbFile=C:\Work\repos\GenericAB\poc_communication_matrix\Zonal_Controller_FL\DBC_ZC_FL_CAN_3.dbc  MsgList=AB_Door_FL_PRV_CAN_Msg_RX1  MsgName=AB_Door_FL_PRV_CAN_Msg_RX1  MsgIDType=Standard (11-bit identifier)  MsgIdentifier=2  MsgLength=8  SignalInfo={'AmpBoard_PRV_CAN_Msg_RX1_Alive','8','4','BE','unsigned','Standard','0','1','0','0','14';'AmpBoard_PRV_CAN_Msg_RX1_CRC','0','8','BE','unsigned','Standard','0','1','0','0','255';'Half_H_Bridge_11_En','44','2','LE','unsigned','Standard','0','1','0','0','3';'LED_En_01','48','2','LE','unsigned','Standard','0','1','0','0','3';'LED_En_02','50','2','LE','unsigned','Standard','0','1','0','0','3';'LED_En_03','52','2','LE','unsigned','Standard','0','1','0','0','3';'LED_En_05','56','2','LE','unsigned','Standard','0','1','0','0','3';'LED_En_06','58','2','LE','unsigned','Standard','0','1','0','0','3';'MirrorGlasAdjustAzimuthLeHa','28','2','LE','unsigned','Standard','0','1','0','0','3';'MirrorGlasAdjustElevationLeHa','30','2','LE','unsigned','Standard','0','1','0','0','3';'OsmCargoLightLeHa','26','2','LE','unsigned','Standard','0','1','0','0','3';'OsmCommonLeHa','24','2','LE','unsigned','Standard','0','1','0','0','3';'OsmHeaterLeHa','42','2','LE','unsigned','Standard','0','1','0','0','3';'OsmLaneChangeAssistLeHa','54','2','LE','unsigned','Standard','0','1','0','0','3';'OsmTaskLightLeHa','46','2','LE','unsigned','Standard','0','1','0','0','3';'OsmTurnSignalLeHa','36','2','LE','unsigned','Standard','0','1','0','0','3';'PowerFoldInLeHa','34','2','LE','unsigned','Standard','0','1','0','0','3';'PowerFoldOutLeHa','32','2','LE','unsigned','Standard','0','1','0','0','3';'PuddleLampLeHa','38','2','LE','unsigned','Standard','0','1','0','0','3';'SideMarkerLampLeHa','40','2','LE','unsigned','Standard','0','1','0','0','3'}  IDPort=off  TimestampPort=off  ErrorPort=off  RemotePort=off  LengthPort=off  StatusPort=off  ApplyMinMax=off
      settings: SourceProductBaseCode=ME,XP,VN  DataFormat=CANdb specified signals
  Data Type Conversion : DataTypeConversion
  Data Type Conversion{1..4,6..7} (6 alike) : DataTypeConversion  OutDataTypeStr=uint8
  Fold_Unfold : Subsystem
  LED1DR_PWM : Subsystem
  LED2DR_PWM : Subsystem
  LED3DR_PWM : Subsystem
  LED4DR_PWM : Subsystem
  LED5DR_PWM : Subsystem
  LED6DR_PWM : Subsystem
  Motor4 : Subsystem
  Motor5 : Subsystem
  Motor6 : Subsystem
  Mux : Mux  Inputs=6
  Subsystem : Subsystem
  Subsystem1 : Subsystem
  Terminator : Terminator
  Terminator48 : Terminator
  Motor : Outport
  RX1_Alive : Outport  Port=2
  wires:
  [Half_H_Bridge_08_En] -> Subsystem/8(Half_H_Bridge_08_En_In)
  Data Type Conversion4/1 -> [LED_En_02]
  Data Type Conversion7/1 -> [LED_En_06]
  [Half_H_Bridge_10_En] -> Subsystem/10(Half_H_Bridge_10_En_In)
  [LED_En_04] -> LED4DR_PWM/1(In1)
  [Half_H_Bridge_09_En] -> Subsystem/9(Half_H_Bridge_09_En_In)
  CAN Unpack1/17 -> [Half_H_Bridge_06_En]
  Subsystem/5(Half_H_Bridge_05_En) -> Fold_Unfold/1(Input)
  CAN Unpack1/12 -> [Half_H_Bridge_01_En]
  [LED_En_02] -> LED2DR_PWM/1(In1)
  [Half_H_Bridge_7_En] -> Subsystem/7(Half_H_Bridge_07_En_In)
  CAN Unpack1/6 -> Data Type Conversion3/1
  CAN Unpack1/18 -> [Half_H_Bridge_05_En]
  Motor5/1(Motor) -> Mux/5
  CAN Unpack1/3 -> [Half_H_Bridge_11_En]
  [Half_H_Bridge_02_En] -> Subsystem/2(Half_H_Bridge_02_En_In)
  CAN Unpack1/20 -> [Half_H_Bridge_09_En]
  [Half_H_Bridge_04_En] -> Subsystem/4(Half_H_Bridge_04_En_In)
  Motor4/1(Motor) -> Mux/4
  Data/1 -> CAN Pack1/1
  CAN Unpack1/4 -> Data Type Conversion6/1
  Data Type Conversion/1 -> Motor/1
  Data Type Conversion2/1 -> [LED_En_04]
  CAN Unpack1/14 -> Data Type Conversion2/1
  Data Type Conversion1/1 -> [LED_En_05]
  Motor6/1(Motor) -> Mux/6
  Subsystem1/1(Motor4) -> Mux/1
  [LED_En_05] -> LED5DR_PWM/1(In1)
  Data Type Conversion3/1 -> [LED_En_03]
  [Half_H_Bridge_05_En] -> Subsystem/5(Half_H_Bridge_05_En_In)
  [LED_En_03] -> LED3DR_PWM/1(In1)
  [Half_H_Bridge_11_En] -> Subsystem/11(Half_H_Bridge_11_En_In)
  [LED_En_01] -> LED1DR_PWM/1(In1)
  Fold_Unfold/1(Motor) -> Mux/3
  Subsystem/4(Half_H_Bridge_04_En) -> Subsystem1/3(up_down)
  [Half_H_Bridge_01_En] -> Subsystem/1(Half_H_Bridge_01_En_In)
  CAN Unpack1/7 -> Data Type Conversion1/1
  [LED_En_06] -> LED6DR_PWM/1(In1)
  Subsystem/3(Half_H_Bridge_03_En) -> Subsystem1/2(right_left)
  Subsystem1/2(Motor5) -> Mux/2
  Subsystem/2(Half_H_Bridge_02_En) -> Terminator/1
  CAN Unpack1/16 -> [Half_H_Bridge_7_En]
  Subsystem/8(Half_H_Bridge_08_En) -> Motor4/2(Input1)
  CAN Unpack1/9 -> [Half_H_Bridge_03_En]
  Subsystem/1(Half_H_Bridge_01_En) -> Subsystem1/1(mirror_common)
  CAN Pack1/1 -> CAN Unpack1/1
  [Half_H_Bridge_06_En] -> Subsystem/6(Half_H_Bridge_06_En_In)
  CAN Unpack1/1 -> RX1_Alive/1
  CAN Unpack1/13 -> [Half_H_Bridge_10_En]
  Mux/1 -> Data Type Conversion/1
  CAN Unpack1/2 -> Terminator48/1
  Data Type Conversion6/1 -> [LED_En_01]
  Subsystem/10(Half_H_Bridge_10_En) -> Motor5/2(Heating)
  [Half_H_Bridge_03_En] -> Subsystem/3(Half_H_Bridge_03_En_In)
  Subsystem/7(Half_H_Bridge_07_En) -> Motor4/1(Input)
  Subsystem/12(Half_H_Bridge_12_En) -> Motor6/2(Input1)
  Subsystem/9(Half_H_Bridge_09_En) -> Motor5/1(Input)
  CAN Unpack1/11 -> [Half_H_Bridge_02_En]
  CAN Unpack1/5 -> Data Type Conversion4/1
  Subsystem/6(Half_H_Bridge_06_En) -> Fold_Unfold/2(Input1)
  CAN Unpack1/8 -> Data Type Conversion7/1
  [Half_H_Bridge_12_En] -> Subsystem/12(Half_H_Bridge_12_En_In)
  CAN Unpack1/10 -> [Half_H_Bridge_04_En]
  CAN Unpack1/19 -> [Half_H_Bridge_08_En]
  Subsystem/11(Half_H_Bridge_11_En) -> Motor6/1(Input)
  CAN Unpack1/15 -> [Half_H_Bridge_12_En]

== system amplifierboard/Digital_Input_Capture/Debounce1 ==
  In1 : Inport
  Add : Sum
  Divide : Product  Inputs=*/
  Init_Val : Constant  OutDataTypeStr=uint16
  Relational Operator : RelationalOperator  Operator=~=  OutDataTypeStr=boolean  RndMeth=Simplest
  Relational Operator1 : RelationalOperator  OutDataTypeStr=boolean  RndMeth=Simplest
  Reset_Val : Constant  Value=0  OutDataTypeStr=uint16
  Switch : Switch  Criteria=u2 ~= 0
  Threshold_Value : Constant  Value=Threshold_Value
  Time_Div : Constant  Value=10  OutDataTypeStr=uint8
  Tolerant_Time : Constant  Value=Tolerant_Time
  Unit Delay : UnitDelay  SampleTime=-1  HasFrameUpgradeWarning=on
  Out1 : Outport
  wires:
  Init_Val/1 -> Add/2
  Reset_Val/1 -> Switch/3
  Threshold_Value/1 -> Relational Operator/2
  Add/1 -> Switch/1
  Unit Delay/1 -> Add/1
  Tolerant_Time/1 -> Divide/1
  Relational Operator/1 -> Switch/2
  Time_Div/1 -> Divide/2
  Divide/1 -> Relational Operator1/2
  Switch/1 -> Relational Operator1/1, Unit Delay/1
  In1/1 -> Relational Operator/1
  Relational Operator1/1 -> Out1/1

== system amplifierboard/Digital_Input_Capture/InvChldLck ==
  In : Inport
  Enumerated Constant2 : simulink/Sources/Enumerated Constant  OutDataTypeStr=Enum: PWRWNDW_CHDLCK  Value=PWRWNDW_CHDLCK.PWRWNDW_CHDLCK_HIGH  SampleTime=inf
  Enumerated Constant3 : simulink/Sources/Enumerated Constant  OutDataTypeStr=Enum: PWRWNDW_CHDLCK  Value=PWRWNDW_CHDLCK.PWRWNDW_CHDLCK_LOW  SampleTime=inf
  Logical Operator1 : Logic  AllPortsSameDT=off  OutDataTypeStr=boolean
  Logical Operator6 : Logic  Operator=XOR  AllPortsSameDT=off  OutDataTypeStr=boolean
  Logical Operator7 : Logic  Operator=NOT  AllPortsSameDT=off  OutDataTypeStr=boolean
  Switch3 : Switch  Criteria=u2 ~= 0
  Unit Delay1 : UnitDelay  SampleTime=-1  HasFrameUpgradeWarning=on
  Unit Delay5 : UnitDelay  SampleTime=-1  HasFrameUpgradeWarning=on
  ChildLock : Outport
  wires:
  Unit Delay1/1 -> Logical Operator1/2
  In/1 -> Unit Delay1/1, Logical Operator7/1
  Unit Delay5/1 -> Logical Operator6/2
  Logical Operator1/1 -> Logical Operator6/1
  Logical Operator6/1 -> Unit Delay5/1, Switch3/2
  Enumerated Constant2/1 -> Switch3/1
  Switch3/1 -> ChildLock/1
  Enumerated Constant3/1 -> Switch3/3
  Logical Operator7/1 -> Logical Operator1/1

== system amplifierboard/HALL_Input_Capture/HEEvents ==
  Function-Call Generator : simulink/Ports & Subsystems/Function-Call Generator  sample_time=-1  numberOfIterations=1  DisallowWideOutput=off
  HE1 : mbd_s32k1xx_ec_toolbox/GPIO Blocks/Digital_Input_ISR  gpio_pin=PTC12: [PTC12 | Port C I/O]  irqc=on rising-edge  prio=15
  HE2 : mbd_s32k1xx_ec_toolbox/GPIO Blocks/Digital_Input_ISR  gpio_pin=PTE10: [PTE10 | Port E I/O]  irqc=on rising-edge  prio=15
  HE3 : mbd_s32k1xx_ec_toolbox/GPIO Blocks/Digital_Input_ISR  gpio_pin=PTD10: [PTD10 | Port D I/O]  irqc=on rising-edge  prio=15
  HE4 : mbd_s32k1xx_ec_toolbox/GPIO Blocks/Digital_Input_ISR  gpio_pin=PTD5: [PTD5 | Port D I/O]  irqc=on rising-edge  prio=15
  HE5 : mbd_s32k1xx_ec_toolbox/GPIO Blocks/Digital_Input_ISR  gpio_pin=PTE15: [PTE15 | Port E I/O]  irqc=on rising-edge  prio=15
  HE6 : mbd_s32k1xx_ec_toolbox/GPIO Blocks/Digital_Input_ISR  gpio_pin=PTE8: [PTE8 | Port E I/O]  irqc=on rising-edge  prio=15
  HE7 : mbd_s32k1xx_ec_toolbox/GPIO Blocks/Digital_Input_ISR  gpio_pin=PTE7: [PTE7 | Port E I/O]  irqc=on rising-edge  prio=15
  HE8 : mbd_s32k1xx_ec_toolbox/GPIO Blocks/Digital_Input_ISR  gpio_pin=PTE4: [PTE4 | Port E I/O]  irqc=on rising-edge  prio=15
  Mux : Mux  Inputs=9
  Events : Outport
  wires:
  Mux/1 -> Events/1
  HE6/1 -> Mux/6
  HE5/1 -> Mux/5
  HE4/1 -> Mux/4
  HE3/1 -> Mux/3
  HE2/1 -> Mux/2
  HE1/1 -> Mux/1
  Function-Call Generator/1 -> Mux/9
  HE7/1 -> Mux/7
  HE8/1 -> Mux/8

== system amplifierboard/Initialization- Memory Defines/Generate_Data ==
  Constant2 : Constant  Value=3  OutDataTypeStr=uint8
  Constant{3,5..6,8} (4 alike) : Constant  Value=2  OutDataTypeStr=uint8
  Constant4 : Constant  OutDataTypeStr=uint8
  Constant7 : Constant  OutDataTypeStr=uint8
  Data Store Read1 : DataStoreRead  DataStoreName=data
  Mux : Mux  Inputs=8
  Width : Width  DataType=uint8
  Data : Outport
  Length : Outport  Port=2
  wires:
  Mux/1 -> Width/1, Data/1
  Constant2/1 -> Mux/1
  Constant3/1 -> Mux/2
  Constant5/1 -> Mux/4
  Data Store Read1/1 -> Mux/5
  Constant4/1 -> Mux/3
  Constant6/1 -> Mux/6
  Constant7/1 -> Mux/7
  Constant8/1 -> Mux/8
  Width/1 -> Length/1

== system amplifierboard/Initialization- Memory Defines/Generate_Data1 ==
  Constant2 : Constant  Value=3  OutDataTypeStr=uint8
  Constant{3,5..6,8} (4 alike) : Constant  Value=2  OutDataTypeStr=uint8
  Constant4 : Constant  OutDataTypeStr=uint8
  Constant7 : Constant  OutDataTypeStr=uint8
  Data Store Read1 : DataStoreRead  DataStoreName=data1
  Mux : Mux  Inputs=8
  Width : Width  DataType=uint8
  Data : Outport
  Length : Outport  Port=2
  wires:
  Mux/1 -> Width/1, Data/1
  Constant2/1 -> Mux/1
  Constant3/1 -> Mux/2
  Constant5/1 -> Mux/4
  Data Store Read1/1 -> Mux/5
  Constant4/1 -> Mux/3
  Constant6/1 -> Mux/6
  Constant7/1 -> Mux/7
  Constant8/1 -> Mux/8
  Width/1 -> Length/1
